simulink model "sim2"  (R2023b)
settings: Solver=VariableStepAuto  StartTime=0.0  StopTime=20  RelTol=1e-3
model workspace (MAT data in the model file):
  b = Simulink.Parameter
  b.Value = 0.1
  b.DataType = 'auto'
  b.Complexity = 'real'
  b.Dimensions = [1 1]
  g = Simulink.Parameter
  g.Value = 9.8
  g.DataType = 'auto'
  g.Complexity = 'real'
  g.Dimensions = [1 1]
  l = Simulink.Parameter
  l.Value = 0.7
  l.DataType = 'auto'
  l.Complexity = 'real'
  l.Dimensions = [1 1]
  m = Simulink.Parameter
  m.Value = 0.2
  m.DataType = 'auto'
  m.Complexity = 'real'
  m.Dimensions = [1 1]
settings Model: Creator=anura  LastModifiedBy=anura
settings DataIOCC: ReturnWorkspaceOutputs=off

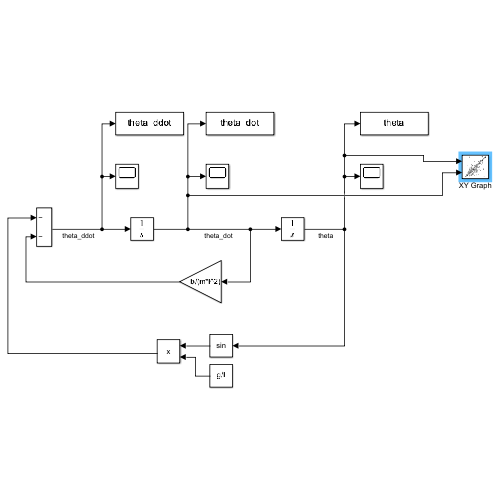
[thumbnail: Simulink's stored preview of the top-level diagram]
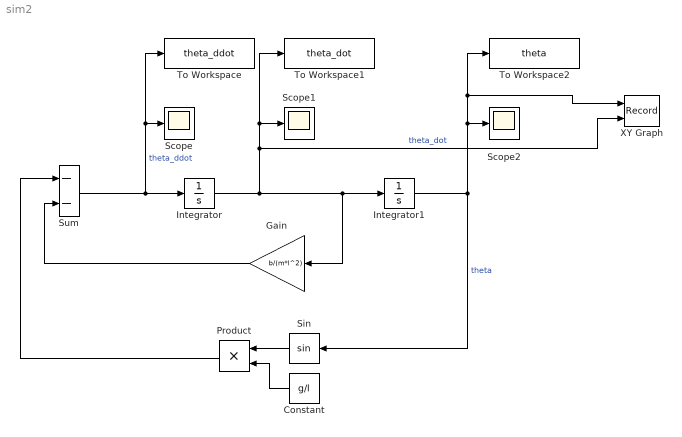
== system sim2 ==
  Constant : Constant  Value=g/l
  Gain : Gain  Gain=b/(m*l^2)
  Integrator : Integrator
  Integrator1 : Integrator  InitialCondition=pi+0.1
  Product : Product
  Scope : Scope
  Scope1 : Scope
  Scope2 : Scope
  Sin : Trigonometry
  Sum : Sum  Inputs=--
  To Workspace : ToWorkspace  VariableName=theta_ddot  SampleTime=-1
  To Workspace1 : ToWorkspace  VariableName=theta_dot  SampleTime=-1
  To Workspace2 : ToWorkspace  VariableName=theta  SampleTime=-1
  XY Graph : Record  FileSettingsInternal="{\"entries\":[{\"content\":{\"excelSettings\":{\"content\":{},\"type\":\"Streamout.ExcelSettings\"}},\"type\":\"Streamout.FileSettingStorage\",\"uuid\":\"\"}],\"packageUris\":[\"http:\\/\\/schema.mathworks.com\\/mf0\\/streamout_blocks\\/R2020a\"],\"version\":\"1.0\"}"  Layout=[1 1]  SignalsInternal="{\"entries\":[{\"content\":{\"signals\":[{\"content\":{\"blockPath\":[],\"dimensions\":[1],\"domain\":\"\",\"lineColor\":\"#a2142f\",\"plots\":[1],\"port\":1,\"sid\":[\"\"],\"signalID\":28,\"signalName\":\"theta\"},\"type\":\"RecordBlkView.Signal\",\"uuid\":\"\"},{\"content\":{\"blockPath\":[],\"dimensions\":[1],\"domain\":\"\",\"lineColor\":\"#139fff\",\"plots\":[1],\"port\":2,\"sid\":[\"\"],\"signalID\":32,\"signalName\":\"theta_dot\"},\"type\":\"RecordBlkView.Signal\",\"uuid\":\"\"}]},\"type\":\"RecordBlkView.InputSignals\",\"uuid\":\"\"}],\"packageUris\":[\"http:\\/\\/schema.mathworks.com\\/mf0\\/streamout_blocks\\/R2020a\"],\"version\":\"1.0\"}"  VisualizationBindings="{\"xyplotplugin\":{\"info\":[{\"series\":[{\"bindingParametersList\":[{\"parameter\":\"X-Axis\",\"signalID\":28,\"signalName\":\"theta\"},{\"parameter\":\"Y-Axis\",\"signalID\":32,\"signalName\":\"theta_dot\"}],\"seriesID\":36373}],\"subplotID\":1}]}}"  CompatibilityTag=XY
  wires:
  Integrator/1 -> XY Graph/2, To Workspace1/1, Scope1/1, Gain/1, Integrator1/1  "theta_dot"
  Sum/1 -> To Workspace/1, Scope/1, Integrator/1  "theta_ddot"
  Gain/1 -> Sum/2
  Integrator1/1 -> Sin/1, XY Graph/1, To Workspace2/1, Scope2/1  "theta"
  Product/1 -> Sum/1
  Sin/1 -> Product/1
  Constant/1 -> Product/2
